simulink model "MassaMolaVarianciaTempo"  (Simulink 7.5)
settings: Solver=ode45  StartTime=0.0  StopTime=200  RelTol=1e-3
settings Model: Creator=Leonardo  LastModifiedBy=Leo

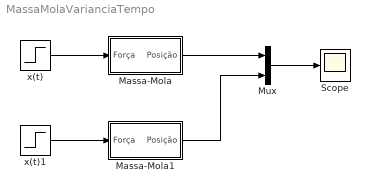
== system MassaMolaVarianciaTempo ==
  Massa-Mola : Subsystem
  Massa-Mola1 : Subsystem
  Mux : Mux  Inputs=2
  Scope : Scope
      settings: TimeRange=100  YMin=0  YMax=1
  x(t) : Step  Time=0  After=50  SampleTime=0  ZeroCross=off
  x(t)1 : Step  Time=100  After=50  SampleTime=0  ZeroCross=off
  wires:
  x(t)/1 -> Massa-Mola/1(Força)
  Mux/1 -> Scope/1
  Massa-Mola/1(Posição) -> Mux/1
  Massa-Mola1/1(Posição) -> Mux/2
  x(t)1/1 -> Massa-Mola1/1(Força)

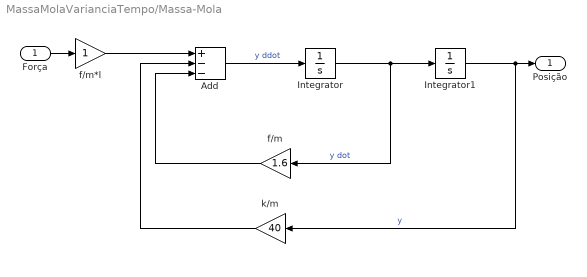
== system MassaMolaVarianciaTempo/Massa-Mola ==
  Força : Inport
  Add : Sum  Inputs=+--
  Integrator : Integrator
  Integrator1 : Integrator
  f/m : Gain  Gain=1.6
  f/m*l : Gain
  k/m : Gain  Gain=40
  Posição : Outport
  wires:
  Integrator/1 -> Integrator1/1, f/m/1  "y dot"
  Add/1 -> Integrator/1  "y ddot"
  Integrator1/1 -> Posição/1, k/m/1  "y"
  k/m/1 -> Add/2
  f/m/1 -> Add/3
  f/m*l/1 -> Add/1
  Força/1 -> f/m*l/1

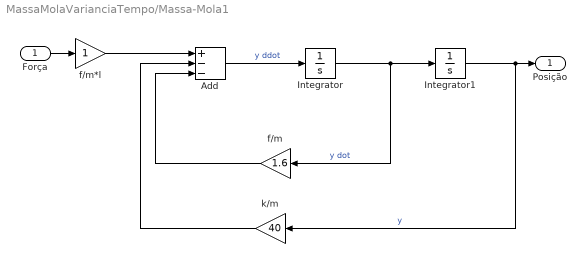
== system MassaMolaVarianciaTempo/Massa-Mola1 ==
  Força : Inport
  Add : Sum  Inputs=+--
  Integrator : Integrator
  Integrator1 : Integrator
  f/m : Gain  Gain=1.6
  f/m*l : Gain
  k/m : Gain  Gain=40
  Posição : Outport
  wires:
  Integrator/1 -> Integrator1/1, f/m/1  "y dot"
  Add/1 -> Integrator/1  "y ddot"
  Integrator1/1 -> Posição/1, k/m/1  "y"
  k/m/1 -> Add/2
  f/m/1 -> Add/3
  f/m*l/1 -> Add/1
  Força/1 -> f/m*l/1
